simulink model "Stoppuhr"  (R2022a)
settings: Solver=ode3  StartTime=0.0  StopTime=10.0  FixedStep=0.01  RelTol=1e-3  EnableMultiTasking=on
settings Model: Creator=60251  LastModifiedBy=yufu
settings SolverCC: AlgebraicLoopSolver=TrustRegion
settings DebuggingCC: UnconnectedInputMsg=warning  UnconnectedOutputMsg=warning  UnconnectedLineMsg=warning  SFMachineParentedDataDiag=warning
settings RTWCC: DLArmComputeVersion=19.05

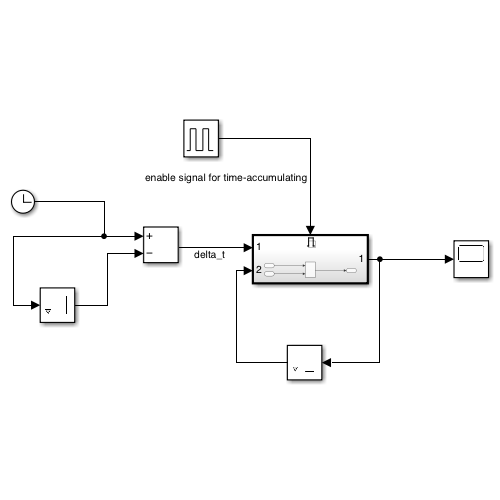
[thumbnail: Simulink's stored preview of the top-level diagram]
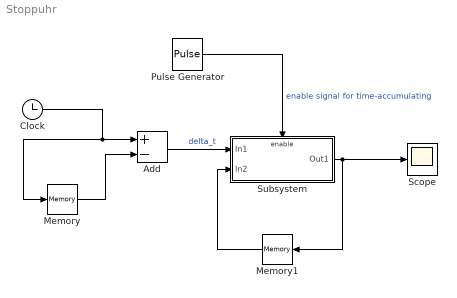
== system Stoppuhr ==
  Add : Sum  Inputs=+-
  Clock : Clock
  Memory : Memory  InheritSampleTime=on
  Memory1 : Memory  InheritSampleTime=on
  Pulse Generator : DiscretePulseGenerator  PulseType=Time based  PulseWidth=50
  Scope : Scope
  Subsystem : Subsystem
  wires:
  Pulse Generator/1 -> Subsystem/Enable  "enable signal for time-accumulating"
  Subsystem/1(Out1) -> Memory1/1, Scope/1
  Clock/1 -> Memory/1, Add/1
  Memory/1 -> Add/2
  Add/1 -> Subsystem/1(In1)  "delta_t"
  Memory1/1 -> Subsystem/2(In2)

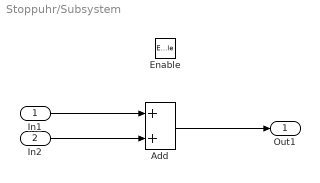
== system Stoppuhr/Subsystem ==
  In1 : Inport
  In2 : Inport  Port=2
  Enable : EnablePort
  Add : Sum
  Out1 : Outport
  wires:
  In1/1 -> Add/1
  Add/1 -> Out1/1
  In2/1 -> Add/2
